simulink model "I_PD_Controller"  (Simulink 10.3)
settings: Solver=VariableStepAuto  StartTime=0.0  StopTime=2  FixedStep=0.001  RelTol=1e-3
undefined symbols (not defined in the file or in its folder): sigbuilder_block
settings Model: Creator=Mertcan  LastModifiedBy=Mertcan
settings SolverCC: AlgebraicLoopSolver=Auto
settings DataIOCC: SaveFormat=Dataset  SignalLoggingSaveFormat=Dataset  ReturnWorkspaceOutputs=on
settings OptimizationCC: ExpressionDepthLimit=128  LifeSpan=auto
settings DebuggingCC: UnderspecifiedInitializationDetection=Simplified  MergeDetectMultiDrivingBlocksExec=error  FcnCallInpInsideContextMsg=error  StateNameClashWarn=none  SFUnexpectedBacktrackingDiag=error  SFNoUnconditionalDefaultTransitionDiag=error  SFExecutionAtInitializationDiag=warning  SFMachineParentedDataDiag=error  ArithmeticOperatorsInVariantConditions=error
settings HardwareCC: ProdBitPerPointer=64  ProdBitPerSizeT=64  ProdBitPerPtrDiffT=64  ProdLargestAtomicFloat=Float  ProdIntDivRoundTo=Zero  ProdEndianess=LittleEndian  ProdWordSize=64  ProdHWDeviceType=Intel->x86-64 (Windows64)
settings ModelReferenceCC: PropagateSignalLabelsOutOfModel=on
settings SFSimCC: SimUseLocalCustomCode=on  CustomCodeUndefinedFunction=FilterOut
settings RTWCC: RTWUseLocalCustomCode=on
settings CodeAppCC: StateflowObjectComments=off
settings GRTTargetCC: TargetLangStandard=C99 (ISO)  CombineOutputUpdateFcns=on  GRTInterface=off
settings ConfigComp: CovMetricSettings=dwe  CovSaveCumulativeToWorkspaceVar=off  CovSaveSingleToWorkspaceVar=off  CovExternalEMLEnable=on

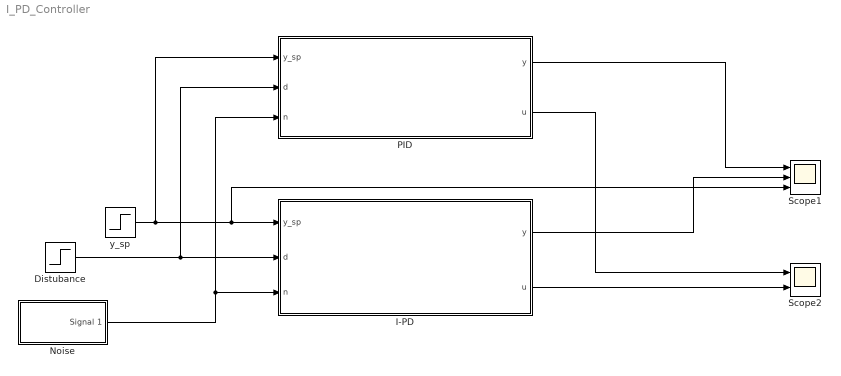
== system I_PD_Controller ==
  Distubance : Step  Time=0.5  After=-1  SampleTime=0
  I-PD : Subsystem
  Noise : Subsystem  Tag=STV Subsys  LoadFcn=sigbuilder_block('load');  StartFcn=sigbuilder_block('start');  StopFcn=sigbuilder_block('stop');  ClipboardFcn=sigbuilder_block('clipboard');  mask(Sigbuilder block){tuvar=[0:10]}
      mask help: Simulink:masks:SigbuilderBlock_MD
      mask init:
      | if ~strcmp(get_param(bdroot(gcbh),'SimulationStatus'),'stopped') tuvar = sigbuilder_block('maskInit'); end
      settings: CopyFcn=sigbuilder_block('copy');  DeleteFcn=sigbuilder_block('delete');  ModelCloseFcn=sigbuilder_block('modelClose');  PreSaveFcn=sigbuilder_block('preSave');  PauseFcn=sigbuilder_block('pause');  ContinueFcn=sigbuilder_block('continue');  NameChangeFcn=sigbuilder_block('namechange');  OpenFcn=sigbuilder_block('open',[6 30 1012.5 447.75 ]);  CloseFcn=sigbuilder_block('close');
      mask Display: plot(0, 0, 100, 100,[2, 2, 32, 32, 2], [68, 8, 8, 68, 68],[32, 2], [38, 38], [32, 19, 2],[53, 60, 44], [32, 17, 17, 2],[16, 16, 31, 31]);txt = getActiveGroup(gcbh);text(2, 100, txt,'verticalAlignment', 'top');
  PID : Subsystem
  Scope1 : Scope  NumInputPorts=3
  Scope2 : Scope  NumInputPorts=2
  y_sp : Step  Time=0  Before=1  SampleTime=0
  wires:
  y_sp/1 -> PID/1(y_sp), Scope1/3, I-PD/1(y_sp)
  Noise/1(Signal 1) -> PID/3(n), I-PD/3(n)
  Distubance/1 -> PID/2(d), I-PD/2(d)
  PID/1(y) -> Scope1/1
  I-PD/1(y) -> Scope1/2
  PID/2(u) -> Scope2/1
  I-PD/2(u) -> Scope2/2

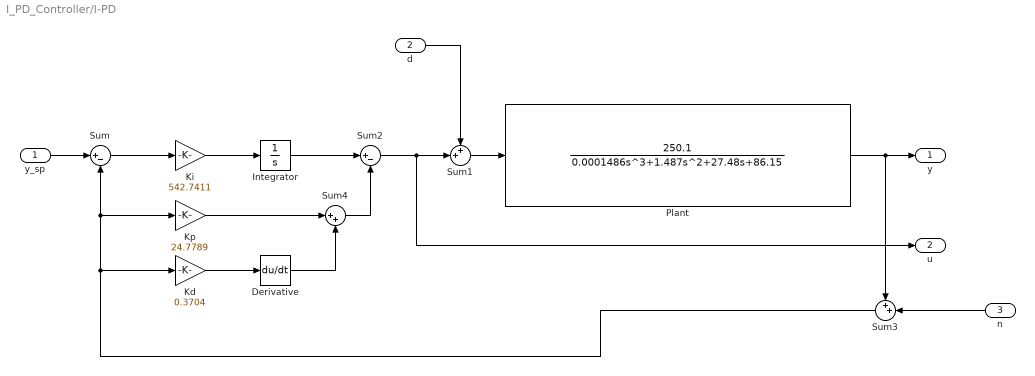
== system I_PD_Controller/I-PD ==
  y_sp : Inport
  d : Inport  Port=2
  n : Inport  Port=3
  Derivative : Derivative
  Integrator : Integrator
  Kd : Gain  Gain=0.3704
  Ki : Gain  Gain=542.7411
  Kp : Gain  Gain=24.7789
  Plant : TransferFcn  Numerator=[250.1]  Denominator=[0.0001486 1.487 27.48 86.15]
  Sum : Sum  Inputs=|+-
  Sum1 : Sum  Inputs=++|
  Sum2 : Sum  Inputs=|+-
  Sum3 : Sum  Inputs=++|
  Sum4 : Sum  Inputs=|++
  y : Outport
  u : Outport  Port=2
  wires:
  Sum2/1 -> Sum1/2, u/1
  Kd/1 -> Derivative/1
  Sum/1 -> Ki/1
  Sum1/1 -> Plant/1
  y_sp/1 -> Sum/1
  Plant/1 -> y/1, Sum3/1
  Ki/1 -> Integrator/1
  n/1 -> Sum3/2
  d/1 -> Sum1/1
  Integrator/1 -> Sum2/1
  Sum3/1 -> Kp/1, Sum/2, Kd/1
  Kp/1 -> Sum4/1
  Sum4/1 -> Sum2/2
  Derivative/1 -> Sum4/2

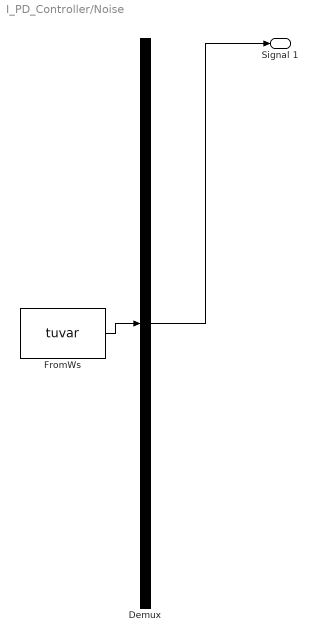
== system I_PD_Controller/Noise ==
  Demux : Demux  Tag=STV Demux  Outputs=1
      settings: DisplayOption=none
  FromWs : FromWorkspace  Tag=STV FromWs  VariableName=tuvar  SigBuilderData=DataTag0  VnvData=DataTag1
      SigBuilderData=|
      | common.afterFinalStr = 'Extrapolate'
      | common.sampleTime = 0
      | dataSet.timeRange = [0 2]
      | dataSet.name = 'Group 1'
      | sbobj.Groups.Name = 'Group 1'
      | sbobj.Groups.Signals.Name = 'Signal 1'
      | sbobj.Groups.Signals.XData = [0 1.5 1.6 1.7 2]
      | sbobj.Groups.Signals.YData = [0 0 0.1 0 0]
      | sbobj.Groups.TimeRange = [0 2]
  Signal 1 : Outport  Tag=STV Outport
  wires:
  Demux/1 -> Signal 1/1
  FromWs/1 -> Demux/1

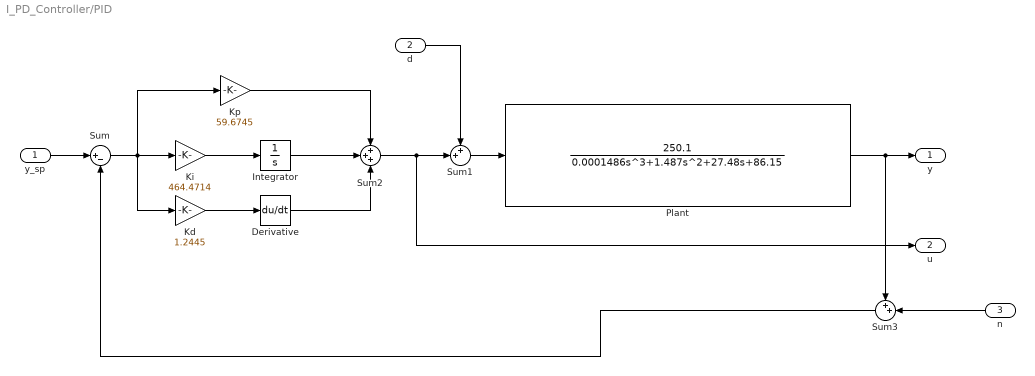
== system I_PD_Controller/PID ==
  y_sp : Inport
  d : Inport  Port=2
  n : Inport  Port=3
  Derivative : Derivative
  Integrator : Integrator
  Kd : Gain  Gain=1.2445
  Ki : Gain  Gain=464.4714
  Kp : Gain  Gain=59.6745
  Plant : TransferFcn  Numerator=[250.1]  Denominator=[0.0001486 1.487 27.48 86.15]
  Sum : Sum  Inputs=|+-
  Sum1 : Sum  Inputs=++|
  Sum2 : Sum  Inputs=+++
  Sum3 : Sum  Inputs=++|
  y : Outport
  u : Outport  Port=2
  wires:
  d/1 -> Sum1/1
  n/1 -> Sum3/2
  Ki/1 -> Integrator/1
  Sum1/1 -> Plant/1
  Sum/1 -> Kd/1, Kp/1, Ki/1
  Plant/1 -> y/1, Sum3/1
  y_sp/1 -> Sum/1
  Sum2/1 -> Sum1/2, u/1
  Kd/1 -> Derivative/1
  Sum3/1 -> Sum/2
  Kp/1 -> Sum2/1
  Integrator/1 -> Sum2/2
  Derivative/1 -> Sum2/3
